simulink model "tr"  (R2023b)
settings: Solver=VariableStepAuto  StartTime=0.0  StopTime=10.0  RelTol=1e-3
libraries: simulink x1
settings Model: Creator=no  LastModifiedBy=no

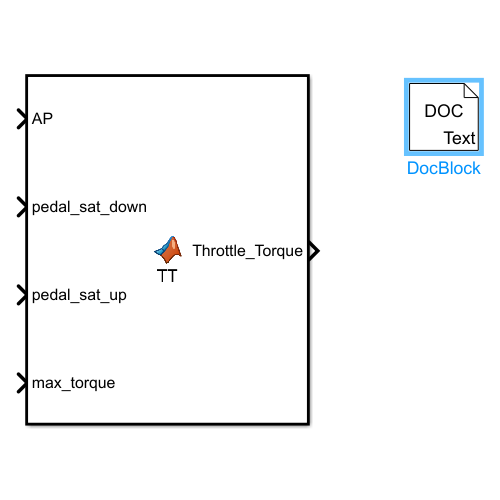
[thumbnail: Simulink's stored preview of the top-level diagram]
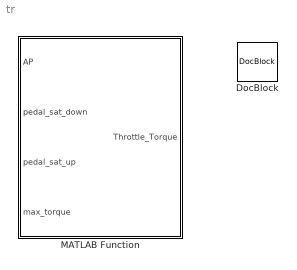
== system tr ==
  DocBlock : simulink/Model-Wide Utilities/DocBlock  DocumentType=Text
      content=|
      | Type your documentation here
  MATLAB Function : MATLAB Function  TreatAsAtomicUnit=on

== matlab function tr/MATLAB Function ==
  data: Throttle_Torque output; AP input; pedal_sat_down input; pedal_sat_up input; max_torque input
function Throttle_Torque  = TT(AP, pedal_sat_down, pedal_sat_up, max_torque)
if AP <= pedal_sat_down %establish the lower deadzone for the throttle pedal
    Throttle_Response = 0;
end
if AP >= pedal_sat_up %establish the higher deadzone for the throttle pedal
    Throttle_Response = 1;
end
if AP >= pedal_sat_down && AP <= pedal_sat_up
    Throttle_Response = (AP/0.6)-(1/3); %evaluate for given input
end
Throttle_Torque = Throttle_Response * max_torque;
end
